simulink model "full_controller_pid"  (R2024a)
settings: Solver=FixedStepAuto  StartTime=0.0  StopTime=SIMTIME  FixedStep=sample_time  RelTol=1e-3
undefined symbols (not defined in the file): desPos, drag_mat, g, Gamma_inv, Jb, Jr, Kd, Kdp, Kdphi, Kdpsi, Kdq, Kdr, Kdx, Kdy, Kip, Kiphi, Kipsi, Kiq, Kir, Kix, Kiy, Kpp, Kpphi, Kppsi, Kpq, Kpr, Kpx, Kpy, Kt, L, m, mot_speeds, psi_des
libraries: matrix_library x2
settings Model: Creator=Lorenzo-Desk  LastModifiedBy=Lorenzo-Desk

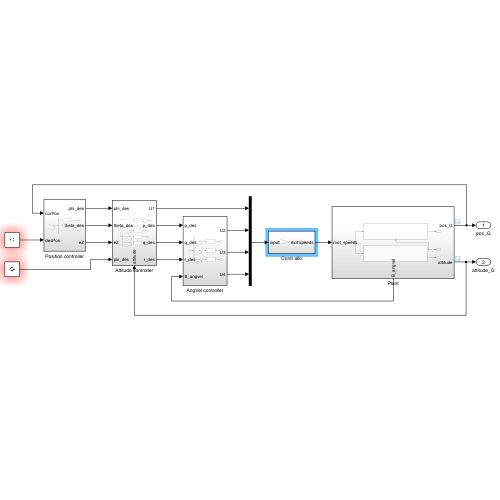
[thumbnail: Simulink's stored preview of the top-level diagram]
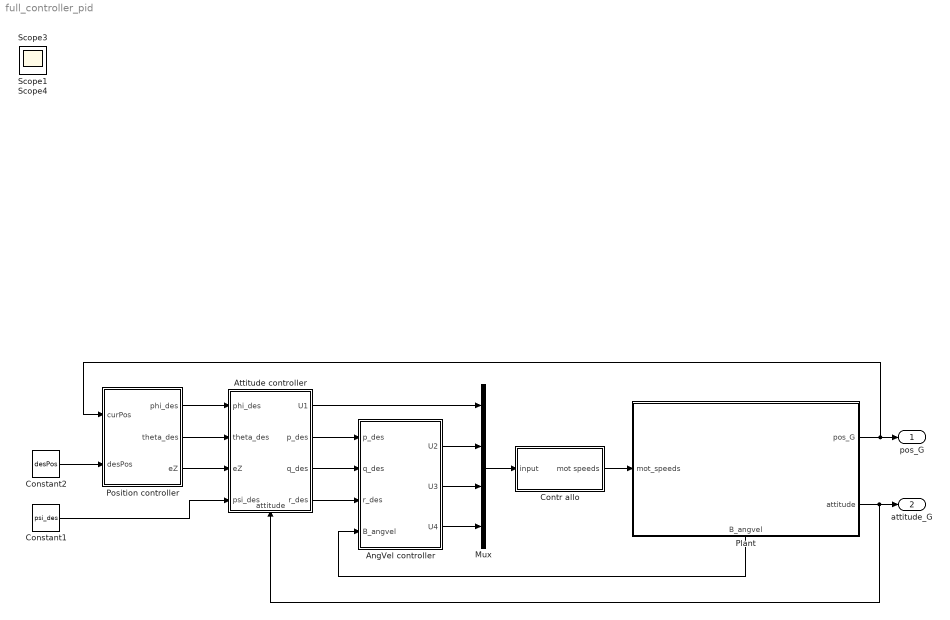
== system full_controller_pid ==
  AngVel controller : Subsystem
  Attitude controller : Subsystem
      settings: PortSchema="{\"entries\":[{\"content\":{\"sides\":[{\"content\":{\"connectorIds\":[\"In1\",\"In2\",\"In3\",\"In4\"]},\"type\":\"ConnectorPlacement.EquallySpacedRectSide\",\"uuid\":\"71281286-38ad-4f2a-91ae-9e6c4e0e30b2\"},{\"content\":{\"connectorIds\":[\"Out1\",\"Out2\",\"Out3\",\"Out4\"],\"side\":\"RIGHT\"},\"type\":\"ConnectorPlacement.EquallySpacedRectSide\",\"uuid\":\"aa649c5f-8758-4d82-8660-affbe0ed2eed\"},{\"content\":{\"side\":\"TOP\"},\"type\":\"ConnectorPlacement.EquallySpacedRectSide\",\"uuid\":\"ccfea5cf-4a16-4d49-8c61-fb0c2c5d9d69\"},{\"content\":{\"connectorIds\":[\"In5\"],\"side\":\"BOTTOM\"},\"type\":\"ConnectorPlacement.EquallySpacedRectSide\",\"uuid\":\"66e9e909-a7d3-4870-b7d3-735590f045d2\"}]},\"type\":\"ConnectorPlacement.EquallySpacedConnector\",\"uuid\":\"1ea574e8-8b7c-489a-8841-cd1e9d9d608b\"}],\"packageUris\":[\"http://schema.mathworks.com/mf0/Connector/R2020b\"],\"version\":\"1.0\"}"
  Constant1 : Constant  Value=psi_des
  Constant2 : Constant  Value=desPos
  Contr allo : Subsystem
  Mux : Mux
  Plant : Subsystem
      settings: PortSchema="{\"entries\":[{\"content\":{\"sides\":[{\"content\":{\"connectorIds\":[\"In1\"]},\"type\":\"ConnectorPlacement.EquallySpacedRectSide\",\"uuid\":\"ebb03a94-9ae7-4e84-aea0-fc42565f8593\"},{\"content\":{\"connectorIds\":[\"Out1\",\"Out2\"],\"side\":\"RIGHT\"},\"type\":\"ConnectorPlacement.EquallySpacedRectSide\",\"uuid\":\"d3caaea2-f7c0-4fac-8e82-acaa745ab632\"},{\"content\":{\"side\":\"TOP\"},\"type\":\"ConnectorPlacement.EquallySpacedRectSide\",\"uuid\":\"5dba95cb-ee08-45fe-863c-0b5d82fe2c1f\"},{\"content\":{\"connectorIds\":[\"Out3\"],\"side\":\"BOTTOM\"},\"type\":\"ConnectorPlacement.EquallySpacedRectSide\",\"uuid\":\"c81cac3f-b299-4c5d-b4ca-e7785434fb4f\"}]},\"type\":\"ConnectorPlacement.EquallySpacedConnector\",\"uuid\":\"99bc8589-d972-4f79-b2a3-5778b2feffef\"}],\"packageUris\":[\"http://schema.mathworks.com/mf0/Connector/R2020b\"],\"version\":\"1.0\"}"
  Position controller : Subsystem
  pos_G : Outport
  attitude_G : Outport  Port=2
  Scope1 : Scope
  Scope3 : Scope
  Scope4 : Scope
  wires:
  Plant/1(pos_G) -> pos_G/1, Position controller/1(curPos)
  Plant/2(attitude) -> Attitude controller/5(attitude), attitude_G/1
  Mux/1 -> Contr allo/1(input)
  Contr allo/1(mot speeds) -> Plant/1(mot_speeds)
  Position controller/1(phi_des) -> Attitude controller/1(phi_des)
  Position controller/2(theta_des) -> Attitude controller/2(theta_des)
  Attitude controller/2(p_des) -> AngVel controller/1(p_des)
  Position controller/3(eZ) -> Attitude controller/3(eZ)
  Constant1/1 -> Attitude controller/4(psi_des)
  Constant2/1 -> Position controller/2(desPos)
  Attitude controller/3(q_des) -> AngVel controller/2(q_des)
  Attitude controller/4(r_des) -> AngVel controller/3(r_des)
  Attitude controller/1(U1) -> Mux/1
  AngVel controller/1(U2) -> Mux/2
  AngVel controller/2(U3) -> Mux/3
  AngVel controller/3(U4) -> Mux/4
  Plant/3(B_angvel) -> AngVel controller/4(B_angvel)

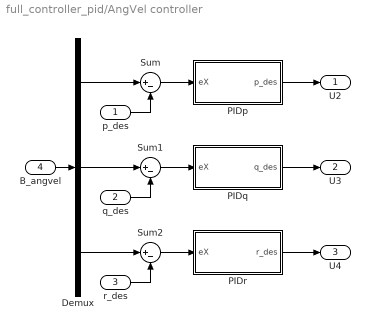
== system full_controller_pid/AngVel controller ==
  p_des : Inport
  q_des : Inport  Port=2
  r_des : Inport  Port=3
  B_angvel : Inport  Port=4
  Demux : Demux  Outputs=3
  PIDp : Subsystem
  PIDq : Subsystem
  PIDr : Subsystem
  Sum : Sum  Inputs=|+-
  Sum1 : Sum  Inputs=|+-
  Sum2 : Sum  Inputs=|+-
  U2 : Outport
  U3 : Outport  Port=2
  U4 : Outport  Port=3
  wires:
  PIDp/1(p_des) -> U2/1
  PIDq/1(q_des) -> U3/1
  PIDr/1(r_des) -> U4/1
  Sum/1 -> PIDp/1(eX)
  Sum1/1 -> PIDq/1(eX)
  Sum2/1 -> PIDr/1(eX)
  p_des/1 -> Sum/2
  q_des/1 -> Sum1/2
  r_des/1 -> Sum2/2
  B_angvel/1 -> Demux/1
  Demux/1 -> Sum/1
  Demux/2 -> Sum1/1
  Demux/3 -> Sum2/1

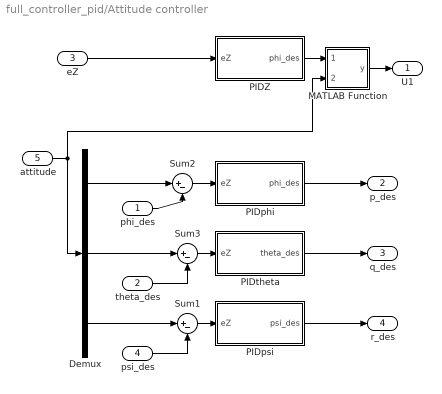
== system full_controller_pid/Attitude controller ==
  phi_des : Inport
  theta_des : Inport  Port=2
  eZ : Inport  Port=3
  psi_des : Inport  Port=4
  attitude : Inport  Port=5
  Demux : Demux  Outputs=3
  MATLAB Function : MATLAB Function  TreatAsAtomicUnit=on
  PIDZ : Subsystem
  PIDphi : Subsystem
  PIDpsi : Subsystem
  PIDtheta : Subsystem
  Sum1 : Sum  Inputs=|+-
  Sum2 : Sum  Inputs=|+-
  Sum3 : Sum  Inputs=|+-
  U1 : Outport
  p_des : Outport  Port=2
  q_des : Outport  Port=3
  r_des : Outport  Port=4
  wires:
  PIDZ/1(phi_des) -> MATLAB Function/1(pidOut)
  MATLAB Function/1(y) -> U1/1
  attitude/1 -> Demux/1, MATLAB Function/2(angles)
  eZ/1 -> PIDZ/1(eZ)
  PIDphi/1(phi_des) -> p_des/1
  PIDtheta/1(theta_des) -> q_des/1
  Sum2/1 -> PIDphi/1(eZ)
  phi_des/1 -> Sum2/2
  Demux/1 -> Sum2/1
  Sum3/1 -> PIDtheta/1(eZ)
  theta_des/1 -> Sum3/2
  Demux/2 -> Sum3/1
  Demux/3 -> Sum1/1
  psi_des/1 -> Sum1/2
  Sum1/1 -> PIDpsi/1(eZ)
  PIDpsi/1(psi_des) -> r_des/1

== system full_controller_pid/Contr allo ==
  input : Inport
  Gain : Gain  Gain=Gamma_inv  Multiplication=Matrix(K*u)
  Gain1 : Gain  Gain=mot_speeds
  SignedSqrt : Sqrt  Operator=signedSqrt  IntermediateResultsDataTypeStr=single
  mot speeds : Outport
  wires:
  input/1 -> Gain/1
  Gain/1 -> SignedSqrt/1
  SignedSqrt/1 -> Gain1/1
  Gain1/1 -> mot speeds/1

== system full_controller_pid/Plant ==
  mot_speeds : Inport
  Rot dyn : Subsystem
  Trans dyn : Subsystem
      settings: PortSchema="{\"entries\":[{\"content\":{\"sides\":[{\"content\":{\"connectorIds\":[\"In1\"]},\"type\":\"ConnectorPlacement.EquallySpacedRectSide\",\"uuid\":\"04ca43f2-6ce4-4aaa-afd3-15a27b70e9d5\"},{\"content\":{\"connectorIds\":[\"Out1\"],\"side\":\"RIGHT\"},\"type\":\"ConnectorPlacement.EquallySpacedRectSide\",\"uuid\":\"cfbeeb74-c76d-4fd7-a96a-210130ba4135\"},{\"content\":{\"side\":\"TOP\"},\"type\":\"ConnectorPlacement.EquallySpacedRectSide\",\"uuid\":\"4de8f8f5-81dc-4bad-a454-bfdfb28428ee\"},{\"content\":{\"connectorIds\":[\"In2\"],\"side\":\"BOTTOM\"},\"type\":\"ConnectorPlacement.EquallySpacedRectSide\",\"uuid\":\"a7fc9bf1-0abd-4a1a-a307-f44f7b0ce4c2\"}]},\"type\":\"ConnectorPlacement.EquallySpacedConnector\",\"uuid\":\"27b8b61f-e2e4-4e1a-8891-32b733733a37\"}],\"packageUris\":[\"http://schema.mathworks.com/mf0/Connector/R2020b\"],\"version\":\"1.0\"}"
  pos_G : Outport
  attitude : Outport  Port=2
  B_angvel : Outport  Port=3
  wires:
  mot_speeds/1 -> Rot dyn/1(mot_speeds), Trans dyn/1(mot_speed)
  Rot dyn/1(attitude) -> attitude/1, Trans dyn/2(attitude)
  Trans dyn/1(pos_G) -> pos_G/1
  Rot dyn/2(B_angvel) -> B_angvel/1

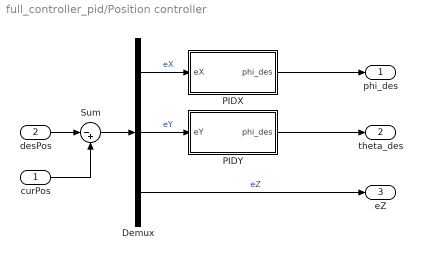
== system full_controller_pid/Position controller ==
  curPos : Inport
  desPos : Inport  Port=2
  Demux : Demux  Outputs=3
  PIDX : Subsystem
  PIDY : Subsystem
  Sum : Sum  Inputs=|-+
  phi_des : Outport
  theta_des : Outport  Port=2
  eZ : Outport  Port=3
  wires:
  PIDX/1(phi_des) -> phi_des/1
  PIDY/1(phi_des) -> theta_des/1
  desPos/1 -> Sum/1
  Sum/1 -> Demux/1
  curPos/1 -> Sum/2
  Demux/1 -> PIDX/1(eX)  "eX"
  Demux/2 -> PIDY/1(eY)  "eY"
  Demux/3 -> eZ/1  "eZ"

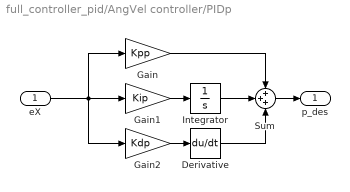
== system full_controller_pid/AngVel controller/PIDp ==
  eX : Inport
  Derivative : Derivative
  Gain : Gain  Gain=Kpp
  Gain1 : Gain  Gain=Kip
  Gain2 : Gain  Gain=Kdp
  Integrator : Integrator
  Sum : Sum  Inputs=+++
  p_des : Outport
  wires:
  Integrator/1 -> Sum/2
  Derivative/1 -> Sum/3
  Gain/1 -> Sum/1
  Sum/1 -> p_des/1
  eX/1 -> Gain/1, Gain1/1, Gain2/1
  Gain1/1 -> Integrator/1
  Gain2/1 -> Derivative/1

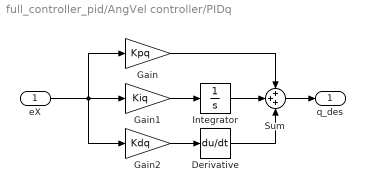
== system full_controller_pid/AngVel controller/PIDq ==
  eX : Inport
  Derivative : Derivative
  Gain : Gain  Gain=Kpq
  Gain1 : Gain  Gain=Kiq
  Gain2 : Gain  Gain=Kdq
  Integrator : Integrator
  Sum : Sum  Inputs=+++
  q_des : Outport
  wires:
  eX/1 -> Gain2/1, Gain1/1, Gain/1
  Sum/1 -> q_des/1
  Gain/1 -> Sum/1
  Derivative/1 -> Sum/3
  Integrator/1 -> Sum/2
  Gain1/1 -> Integrator/1
  Gain2/1 -> Derivative/1

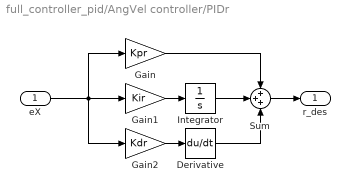
== system full_controller_pid/AngVel controller/PIDr ==
  eX : Inport
  Derivative : Derivative
  Gain : Gain  Gain=Kpr
  Gain1 : Gain  Gain=Kir
  Gain2 : Gain  Gain=Kdr
  Integrator : Integrator
  Sum : Sum  Inputs=+++
  r_des : Outport
  wires:
  Integrator/1 -> Sum/2
  Derivative/1 -> Sum/3
  Gain/1 -> Sum/1
  Sum/1 -> r_des/1
  eX/1 -> Gain/1, Gain1/1, Gain2/1
  Gain1/1 -> Integrator/1
  Gain2/1 -> Derivative/1

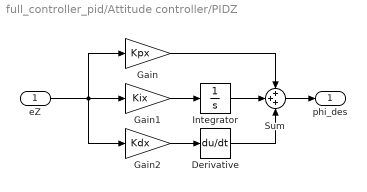
== system full_controller_pid/Attitude controller/PIDZ ==
  eZ : Inport
  Derivative : Derivative
  Gain : Gain  Gain=Kpx
  Gain1 : Gain  Gain=Kix
  Gain2 : Gain  Gain=Kdx
  Integrator : Integrator
  Sum : Sum  Inputs=+++
  phi_des : Outport
  wires:
  Integrator/1 -> Sum/2
  Derivative/1 -> Sum/3
  Gain/1 -> Sum/1
  Sum/1 -> phi_des/1
  eZ/1 -> Gain2/1, Gain1/1, Gain/1
  Gain1/1 -> Integrator/1
  Gain2/1 -> Derivative/1

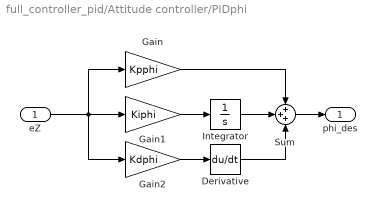
== system full_controller_pid/Attitude controller/PIDphi ==
  eZ : Inport
  Derivative : Derivative
  Gain : Gain  Gain=Kpphi
  Gain1 : Gain  Gain=Kiphi
  Gain2 : Gain  Gain=Kdphi
  Integrator : Integrator
  Sum : Sum  Inputs=+++
  phi_des : Outport
  wires:
  eZ/1 -> Gain2/1, Gain1/1, Gain/1
  Sum/1 -> phi_des/1
  Gain/1 -> Sum/1
  Derivative/1 -> Sum/3
  Integrator/1 -> Sum/2
  Gain1/1 -> Integrator/1
  Gain2/1 -> Derivative/1

== system full_controller_pid/Attitude controller/PIDpsi ==
  eZ : Inport
  Derivative : Derivative
  Gain : Gain  Gain=Kppsi
  Gain1 : Gain  Gain=Kipsi
  Gain2 : Gain  Gain=Kdpsi
  Integrator : Integrator
  Sum : Sum  Inputs=+++
  psi_des : Outport
  wires:
  eZ/1 -> Gain2/1, Gain1/1, Gain/1
  Sum/1 -> psi_des/1
  Gain/1 -> Sum/1
  Derivative/1 -> Sum/3
  Integrator/1 -> Sum/2
  Gain1/1 -> Integrator/1
  Gain2/1 -> Derivative/1

== system full_controller_pid/Attitude controller/PIDtheta ==
  eZ : Inport
  Derivative : Derivative
  Gain : Gain  Gain=Kpphi
  Gain1 : Gain  Gain=Kiphi
  Gain2 : Gain  Gain=Kdphi
  Integrator : Integrator
  Sum : Sum  Inputs=+++
  theta_des : Outport
  wires:
  Integrator/1 -> Sum/2
  Derivative/1 -> Sum/3
  Gain/1 -> Sum/1
  Sum/1 -> theta_des/1
  eZ/1 -> Gain/1, Gain1/1, Gain2/1
  Gain1/1 -> Integrator/1
  Gain2/1 -> Derivative/1

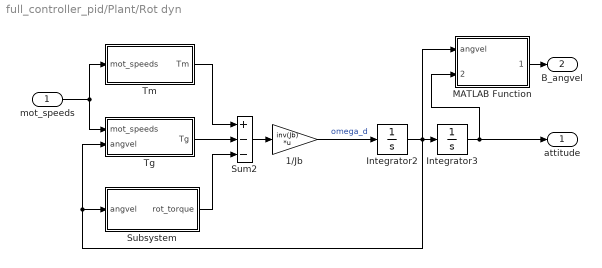
== system full_controller_pid/Plant/Rot dyn ==
  mot_speeds : Inport
  1/Jb : Gain  Gain=inv(Jb)  Multiplication=Matrix(K*u)
  Integrator2 : Integrator
  Integrator3 : Integrator
  MATLAB Function : MATLAB Function  TreatAsAtomicUnit=on
  Subsystem : Subsystem
  Sum2 : Sum  Inputs=+--
  Tg : Subsystem
  Tm : Subsystem
  attitude : Outport
  B_angvel : Outport  Port=2
  wires:
  Subsystem/1(rot_torque) -> Sum2/3
  Sum2/1 -> 1/Jb/1
  Tm/1(Tm) -> Sum2/1
  1/Jb/1 -> Integrator2/1  "omega_d"
  Integrator2/1 -> MATLAB Function/1(angvel), Integrator3/1, Tg/2(angvel), Subsystem/1(angvel)
  Integrator3/1 -> MATLAB Function/2(attitude), attitude/1
  mot_speeds/1 -> Tm/1(mot_speeds), Tg/1(mot_speeds)
  Tg/1(Tg) -> Sum2/2
  MATLAB Function/1(B_angvel) -> B_angvel/1

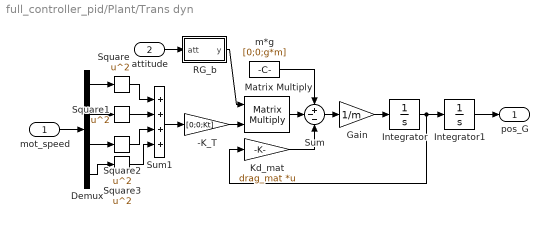
== system full_controller_pid/Plant/Trans dyn ==
  mot_speed : Inport
  attitude : Inport  Port=2
  -K_T : Gain  Gain=[0;0;Kt]
  Demux : Demux
  Gain : Gain  Gain=1/m
  Integrator : Integrator
  Integrator1 : Integrator
  Kd_mat : Gain  Gain=drag_mat  Multiplication=Matrix(K*u)
  Matrix Multiply : Product  Multiplication=Matrix(*)
  RG_b : MATLAB Function  TreatAsAtomicUnit=on
  Square{,1..3} (4 alike) : Math  Operator=square
  Sum : Sum  Inputs=+--
  Sum1 : Sum  Inputs=++++
  m*g : Constant  Value=[0;0;g*m]
  pos_G : Outport
  wires:
  Integrator/1 -> Integrator1/1, Kd_mat/1
  Kd_mat/1 -> Sum/3
  Square/1 -> Sum1/1
  Square1/1 -> Sum1/2
  Square3/1 -> Sum1/4
  Integrator1/1 -> pos_G/1
  Demux/1 -> Square/1
  Demux/3 -> Square2/1
  mot_speed/1 -> Demux/1
  attitude/1 -> RG_b/1(att)
  Sum1/1 -> -K_T/1
  Gain/1 -> Integrator/1
  Square2/1 -> Sum1/3
  Sum/1 -> Gain/1
  -K_T/1 -> Matrix Multiply/2
  Demux/4 -> Square3/1
  Demux/2 -> Square1/1
  Matrix Multiply/1 -> Sum/2
  RG_b/1(y) -> Matrix Multiply/1
  m*g/1 -> Sum/1

== system full_controller_pid/Position controller/PIDX ==
  eX : Inport
  Derivative : Derivative
  Gain : Gain  Gain=Kpx
  Gain1 : Gain  Gain=Kix
  Gain2 : Gain  Gain=Kdx
  Integrator : Integrator
  Sum : Sum  Inputs=+++
  phi_des : Outport
  wires:
  Integrator/1 -> Sum/2
  Derivative/1 -> Sum/3
  Gain/1 -> Sum/1
  Sum/1 -> phi_des/1
  eX/1 -> Gain/1, Gain1/1, Gain2/1
  Gain1/1 -> Integrator/1
  Gain2/1 -> Derivative/1

== system full_controller_pid/Position controller/PIDY ==
  eY : Inport
  Derivative : Derivative
  Gain : Gain  Gain=Kpy
  Gain1 : Gain  Gain=Kiy
  Gain2 : Gain  Gain=Kdy
  Integrator : Integrator
  Sum : Sum  Inputs=+++
  phi_des : Outport
  wires:
  eY/1 -> Gain2/1, Gain1/1, Gain/1
  Sum/1 -> phi_des/1
  Gain/1 -> Sum/1
  Derivative/1 -> Sum/3
  Integrator/1 -> Sum/2
  Gain1/1 -> Integrator/1
  Gain2/1 -> Derivative/1

== system full_controller_pid/Plant/Rot dyn/Subsystem ==
  angvel : Inport
  Cross Product : matrix_library/Cross Product
  Jb : Gain  Gain=Jb  Multiplication=Matrix(K*u)
  rot_torque : Outport
  wires:
  Cross Product/1 -> rot_torque/1
  angvel/1 -> Cross Product/1, Jb/1
  Jb/1 -> Cross Product/2

== system full_controller_pid/Plant/Rot dyn/Tg ==
  mot_speeds : Inport
  angvel : Inport  Port=2
  Cross Product : matrix_library/Cross Product
  Demux : Demux
  Jr : Gain  Gain=[0;0;Jr]
  Sum : Sum  Inputs=+-+-
  Tg : Outport
  wires:
  mot_speeds/1 -> Demux/1
  Demux/4 -> Sum/4
  Demux/1 -> Sum/1
  Demux/2 -> Sum/2
  Demux/3 -> Sum/3
  Sum/1 -> Jr/1
  angvel/1 -> Cross Product/1
  Jr/1 -> Cross Product/2
  Cross Product/1 -> Tg/1

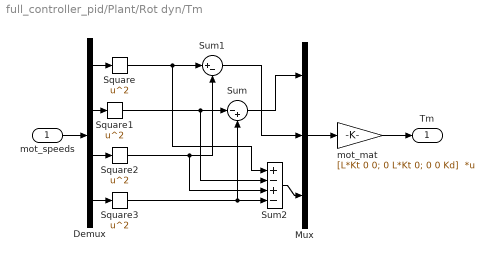
== system full_controller_pid/Plant/Rot dyn/Tm ==
  mot_speeds : Inport
  Demux : Demux
  Mux : Mux  Inputs=3
  Square{,1..3} (4 alike) : Math  Operator=square
  Sum : Sum  Inputs=|-+
  Sum1 : Sum  Inputs=|+-
  Sum2 : Sum  Inputs=+-+-
  mot_mat : Gain  Gain=[L*Kt 0 0; 0 L*Kt 0; 0 0 Kd]  Multiplication=Matrix(K*u)
  Tm : Outport
  wires:
  mot_speeds/1 -> Demux/1
  Demux/1 -> Square/1
  Demux/2 -> Square1/1
  Demux/3 -> Square2/1
  Demux/4 -> Square3/1
  Square3/1 -> Sum2/4, Sum/2
  Square2/1 -> Sum2/3, Sum1/2
  Square/1 -> Sum2/1, Sum1/1
  Mux/1 -> mot_mat/1
  Sum2/1 -> Mux/3
  Square1/1 -> Sum2/2, Sum/1
  mot_mat/1 -> Tm/1
  Sum/1 -> Mux/1
  Sum1/1 -> Mux/2

== matlab function full_controller_pid/Attitude controller/MATLAB Function ==
  data: pidOut input; y output; angles input
function y = fcn(pidOut, angles)
phi = angles(1);
theta = angles(2);
y = 1/(cos(phi)*cos(theta))*pidOut;

== matlab function full_controller_pid/Plant/Rot dyn/MATLAB Function ==
  data: angvel input; attitude input; B_angvel output
function B_angvel = fcn(angvel, attitude)
phi = attitude(1);
theta = attitude(2);
psi = attitude(3);
S = [1 0 -sin(theta);
     0 cos(phi) sin(phi)*cos(theta);
     0 -sin(phi) cos(phi)*cos(theta)];
B_angvel = S*angvel;

== matlab function full_controller_pid/Plant/Trans dyn/RG_b ==
  data: att input; y output
function y = fcn(att)
phi = att(1); theta = att(2); psi = att(3);

y = [cos(psi)*cos(theta)    sin(psi)*cos(theta) -sin(theta);
     cos(psi)*sin(phi)*sin(theta)-cos(phi)*sin(psi) sin(phi)*sin(psi)*sin(theta)+cos(phi)*cos(psi)  cos(theta)*sin(phi);
     cos(phi)*cos(psi)*sin(theta)+sin(phi)*sin(psi) cos(phi)*sin(psi)*sin(theta)-cos(psi)*sin(phi)  cos(phi)*cos(theta)];
